simulink model "sim_regulation"  (R2024b)
settings: Solver=VariableStepAuto  StartTime=0.0  StopTime=T_SIM  MaxStep=0.001  RelTol=1e-3
values from neighbouring files (symbols this model uses):
  control_par = [k_1, k_2, k_3]    [regulation_script.m]    (also in traj_tracking_script.m = [k1, k2,b])
  controller_index = 2    [regulation_script.m]    (also in traj_tracking_script.m = 1)
  d = d_actual    (= 0.1694)    [regulation_script.m]    (also in traj_tracking_script.m = 0.165)
  d_actual = 0.1694    [regulation_script.m]    (also in traj_tracking_script.m = 0.165)
  omega_M = 10    [regulation_script.m]    (also in traj_tracking_script.m = 12)
  q_d = [0;0;0]    [regulation_script.m]
  Q_INIT = [0;-2;pi/2+0.01]    [regulation_script.m]    (also in traj_tracking_script.m = [.2; 0.; pi/2])
  r = r_actual    (= 0.0302)    [regulation_script.m]    (also in traj_tracking_script.m = 0.03)
  r_actual = 0.0302    [regulation_script.m]    (also in traj_tracking_script.m = 0.03)
settings Model: Creator=alber  LastModifiedBy=llp
settings RTWCC: GPUComputeCapability=3.5

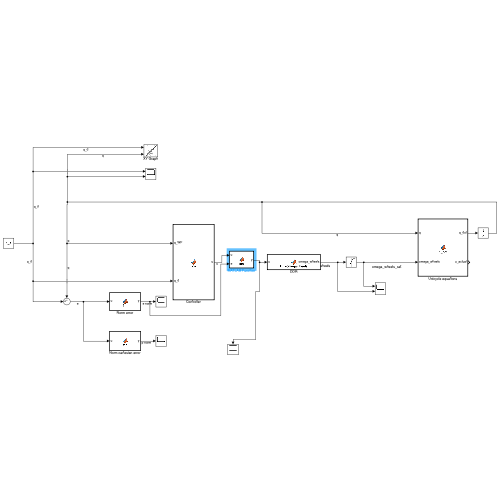
[thumbnail: Simulink's stored preview of the top-level diagram]
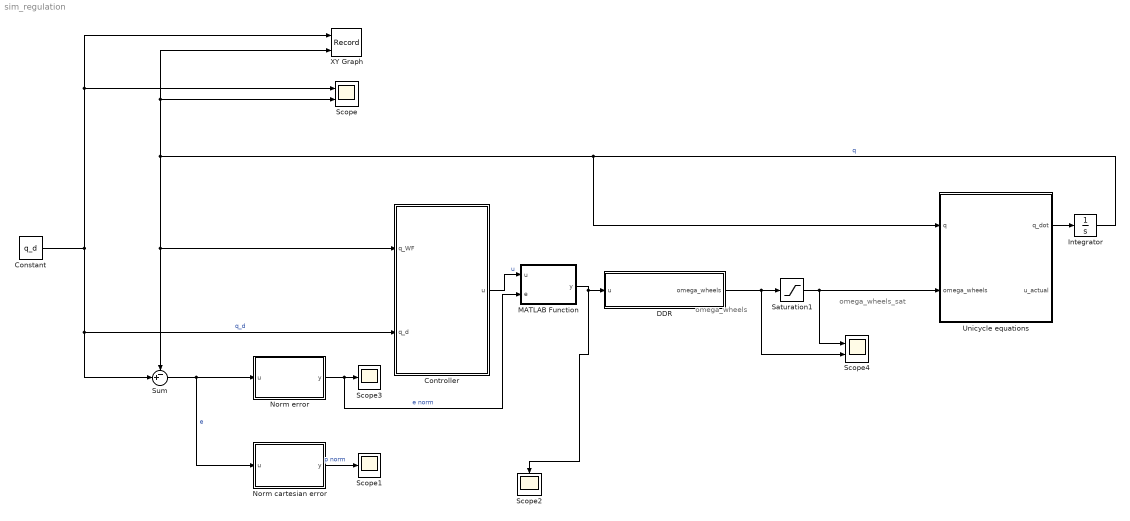
== system sim_regulation ==
  note: omega_wheels_sat
  note: omega_wheels
  Constant : Constant  Value=q_d
  Controller : MATLAB Function  TreatAsAtomicUnit=on
  DDR : MATLAB Function  TreatAsAtomicUnit=on
  Integrator : Integrator  InitialCondition=Q_INIT
  MATLAB Function : MATLAB Function  TreatAsAtomicUnit=on
  Norm cartesian error : MATLAB Function  TreatAsAtomicUnit=on
  Norm error : MATLAB Function  TreatAsAtomicUnit=on
  Saturation1 : Saturate  UpperLimit=omega_M  LowerLimit=-omega_M
  Scope : Scope  NumInputPorts=2
  Scope1 : Scope
  Scope2 : Scope
  Scope3 : Scope
  Scope4 : Scope  NumInputPorts=2
  Sum : Sum  Inputs=-+|
  Unicycle equations : MATLAB Function  TreatAsAtomicUnit=on
  XY Graph : Record  FileSettingsInternal="{\"entries\":[{\"content\":{\"excelSettings\":{\"content\":{},\"type\":\"Streamout.ExcelSettings\"}},\"type\":\"Streamout.FileSettingStorage\",\"uuid\":\"\"}],\"packageUris\":[\"http:\\/\\/schema.mathworks.com\\/mf0\\/streamout_blocks\\/R2020a\"],\"version\":\"1.0\"}"  Layout=[1 1]  SignalsInternal="{\"entries\":[{\"content\":{\"signals\":[{\"content\":{\"blockPath\":[],\"dimensions\":[3,1],\"domain\":\"\",\"hasChildren\":true,\"lineColor\":\"#fe330a\",\"lineWidth\":2,\"port\":2,\"sid\":[\"\"],\"signalID\":1,\"signalName\":\"q\"},\"type\":\"RecordBlkView.Signal\",\"uuid\":\"\"},{\"content\":{\"blockPath\":[],\"channel\":[1,1],\"dimensions\":[3,1],\"domain\":\"\",\"lineColor\":\"#000000\",\"lineStyle\":\"DASH_DOT\",\"parentID\":1,\"plots\":[ 1 ],\"port\":2,\"sid\":[\"\"],\"signalID\":2,\"signalName\":\"q\"},\"type\":\"RecordBlkView.Signal\",\"uuid\":\"\"},{\"content\":{\"blockPath\":[],\"dimensions\":[3],\"domain\":\"\",\"hasChildren\":true,\"lineColor\":\"#0072bd\",\"lineWidth\":2,\"port\":1,\"sid\":[\"\"],\"signalID\":3,\"signalName\":\"q_d\"},\"type\":\"RecordBlkView.Signal\",\"uuid\":\"\"},{\"content\":{\"blockPath\":[],\"channel\":[1],\"dimensions\":[3],\"domain\":\"\",\"lineColor\":\"#d95319\",\"parentID\":3,\"port\":1,\"sid\":[\"\"],\"signalID\":4,\"signalName\":\"q_d\"},\"type\":\"RecordBlkView.Signal\",\"uuid\":\"\"},{\"content\":{\"blockPath\":[],\"channel\":[2,1],\"dimensions\":[3,1],\"domain\":\"\",\"lineColor\":\"#000000\",\"lineStyle\":\"DASH_DOT\",\"parentID\":1,\"plots\":[ 1 ],\"port\":2,\"sid\":[\"\"],\"signalID\":5,\"signalName\":\"q\"},\"type\":\"RecordBlkView.Signal\",\"uuid\":\"\"},{\"content\":{\"blockPath\":[],\"channel\":[3,1],\"dimensions\":[3,1],\"domain\":\"\",\"lineColor\":\"#b746ff\",\"parentID\":1,\"port\":2,\"sid\":[\"\"],\"signalID\":6,\"signalName\":\"q\"},\"type\":\"RecordBlkView.Signal\",\"uuid\":\"\"},{\"content\":{\"blockPath\":[],\"channel\":[2],\"dimensions\":[3],\"domain\":\"\",\"lineColor\":\"#77ac30\",\"parentID\":3,\"port\":1,\"sid\":[\"\"],\"signalID\":7,\"signalName\":\"q_d\"},\"type\":\"RecordBlkView.Signal\",\"uuid\":\"\"},{\"content\":{\"blockPath\":[],\"channel\":[3],\"dimensions\":[3],\"domain\":\"\",\"lineColor\":\"#4dbeee\",\"parentID\":3,\"port\":1,\"sid\":[\"\"],\"signalID\":8,\"signalName\":\"q_d\"},\"type\":\"RecordBlkView.Signal\",\"uuid\":\"\"}]},\"type\":\"RecordBlkView.InputSignals\",\"uuid\":\"\"}],\"packageUris\":[\"http:\\/\\/schema.mathworks.com\\/mf0\\/streamout_blocks\\/R2020a\"],\"version\":\"1.0\"}"  VisualizationBindings="{\"xyplotplugin\":{\"info\":[{\"series\":[{\"bindingParametersList\":[{\"parameter\":\"X-Axis\",\"signalID\":2,\"signalName\":\"q(1,1)\"},{\"parameter\":\"Y-Axis\",\"signalID\":5,\"signalName\":\"q(2,1)\"}],\"seriesID\":0}],\"subplotID\":1}]}}"  CompatibilityTag=XY
  wires:
  Integrator/1 -> Sum/1, Controller/1(q_WF), XY Graph/2, Scope/2, Unicycle equations/1(q)  "q"
  Unicycle equations/1(q_dot) -> Integrator/1
  Constant/1 -> Sum/2, Controller/2(q_d), XY Graph/1, Scope/1  "q_d"
  Sum/1 -> Norm cartesian error/1(u), Norm error/1(u)  "e"
  Controller/1(u) -> MATLAB Function/1(u)  "u"
  Norm cartesian error/1(y) -> Scope1/1  "p norm"
  DDR/1(omega_wheels) -> Saturation1/1, Scope4/2
  Saturation1/1 -> Unicycle equations/2(omega_wheels), Scope4/1
  Norm error/1(y) -> MATLAB Function/2(e), Scope3/1  "e norm"
  MATLAB Function/1(y) -> Scope2/1, DDR/1(u)

== matlab function sim_regulation/Norm cartesian error ==
  data: u input; y output
function y = fcn(u)

y = sqrt(sum(u(1:2).^2));

== matlab function sim_regulation/Unicycle equations ==
  data: q input; omega_wheels input; q_dot output; r_actual parameter; d_actual parameter; u_actual output
function [q_dot, u_actual] = q_dot(q, omega_wheels, r_actual, d_actual)
u_actual = [r_actual/2, r_actual/2;-r_actual/d_actual, r_actual/d_actual]*omega_wheels;
theta = q(3);
q_dot = [[cos(theta), 0];[sin(theta), 0];[0,1]]*u_actual;

== matlab function sim_regulation/Norm error ==
  data: u input; y output
function y = fcn(u)
y = [u(1);u(2); wrapToPi(u(3))];

== matlab function sim_regulation/Controller ==
  data: q_WF input; q_d input; u output; controller_index parameter; control_par parameter
function u = fcn(q_WF, q_d, controller_index, control_par)
% select the controller
k1 = control_par(1);
k2 = control_par(2);
k3 = control_par(3);

xd = q_d(1);
yd = q_d(2);
thetad = q_d(3);

if controller_index == 1
    % cartesian regulator
    % transform q_WF
    x_t = q_WF(1) -xd;
    y_t = q_WF(2)-yd;
    theta = q_WF(3);

    gamma = atan2(y_t,x_t)+pi-theta;

    % compute the input

    v = -k1*(x_t*cos(theta)+y_t*sin(theta));
    omega = k2*gamma;

    u = [v;omega];
else
    % posture regulator
    % transform q_WF
    
    e = q_WF-q_d;

    x_t = cos(thetad)*e(1)+sin(thetad)*e(2);
    y_t = -sin(thetad)*e(1)+cos(thetad)*e(2);
    theta_t = e(3);

    rho = sqrt(x_t^2+y_t^2);
    gamma = atan2(y_t,x_t)+pi-theta_t;
    delta = theta_t +gamma;

    v = k1*rho*cos(gamma);
    omega = k2*gamma + k1 *(sin(gamma)*cos(gamma))/gamma *(gamma+k3*delta);

    % compute pointing error
    u = [v;omega];
end

== matlab function sim_regulation/DDR ==
  data: u input; omega_wheels output; r parameter; d parameter
function omega_wheels = kin2omegawheels(u, r, d)
omega_l = u(1)/r-d/(2*r)*u(2);
omega_r = u(1)/r+d/(2*r)*u(2);
omega_wheels = [omega_l;omega_r];

== matlab function sim_regulation/MATLAB Function ==
  data: u input; y output; e input; tol data_store_memory
function y = fcn(u, e)

e_x = e(1);
e_y = e(2);
e_theta = e(3);

if (e_x < tol & y_x< tol & e_theta<tol)
 y = 0;
else
 y = u;

end
